simulink model "montagemrobo2"  (R2018a)
settings: Solver=VariableStepAuto  StartTime=0.0  StopTime=120  RelTol=1e-3
model workspace: external: MATLAB File C:\Users\Thiago\Documents\1- Faculdade\Robotica\2020.1\TRABALHO\simulink\montagemrobo_DataFile1.m (data not in the file)
values from neighbouring files (symbols this model uses):
  m = [207.61613 346.81729 366.65763 243.34094 10.76884 27.61521 3.40236]    [matlab.mat]
undefined symbols (not defined in the file or in its folder): smiData, X, Y, Z
libraries: sm_lib x61, nesl_utility x7
(part 2 of 2)

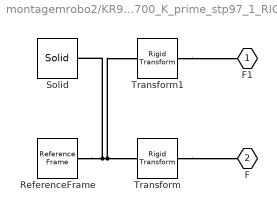
== system montagemrobo2/KR90_R3700_K_prime_stp97_1_RIGID ==
  ReferenceFrame : sm_lib/Frames and Transforms/Reference Frame
  Solid : sm_lib/Body Elements/Solid  InertiaType=Custom  Mass=smiData.Solid(6).mass  MassUnits=kg  CenterOfMass=smiData.Solid(6).CoM  CenterOfMassUnits=mm  MomentsOfInertia=smiData.Solid(6).MoI  MomentsOfInertiaUnits=kg*mm^2  ProductsOfInertia=smiData.Solid(6).PoI  ProductsOfInertiaUnits=kg*mm^2  DensityBased=on  Density=1000  DensityUnits=kg/m^3  DoExposeReferenceFrame=on  SerializedFrames=<Frames/>  GraphicType=FromGeometry  MarkerShape=Sphere  MarkerSize=10  GraphicVisPropType=SimpleVisualProperties  GraphicDiffuseColor=smiData.Solid(6).color  GraphicSpecularColor=[0.5 0.5 0.5 1.0]  GraphicAmbientColor=[0.15 0.15 0.15 1.0]  GraphicEmissiveColor=[0.0 0.0 0.0 1.0]  GraphicShininess=75  GraphicOpacity=smiData.Solid(6).opacity  GeometryShape=FromFile  RectangleSize=[1 1]  RectangleSizeUnits=m  BrickDimensions=[1 1 1]  BrickDimensionUnits=m  CylinderRadius=1  CylinderRadiusUnits=m  CylinderLength=1  CylinderLengthUnits=m  SphereRadius=1  SphereRadiusUnits=m  EllipsoidRadii=[1 1 1]  EllipsoidRadiiUnits=m  ExtrusionCrossSection=[1 1; -1 1; -1 -1; 1 -1]  ExtrusionCrossSectionUnits=m  ExtrusionLength=1  ExtrusionLengthUnits=m  PolygonNumSides=3  PolygonOuterRadius=1  PolygonOuterRadiusUnits=m  ExtGeomFileType=STEP  ExtGeomFileName=KR90_R3700_K_prime.stp[97]_Valor predeterminado_sldprt.STEP  ExtGeomFileUnits=m  RevolutionCrossSection=[1 1; 1 -1; 2 -1; 2 1]  RevolutionCrossSectionUnits=m  RevolutionExtent=Full  RevolutionAngle=180  RevolutionAngleUnits=deg
  Transform : sm_lib/Frames and Transforms/Rigid Transform  TranslationMethod=Cartesian  TranslationStandardOffset=0  TranslationLengthUnit=mm  TranslationStandardAxis=+Z  TranslationCartesianOffset=smiData.RigidTransform(4).translation  TranslationROffset=0  TranslationROffsetUnits=m  TranslationZOffset=0  TranslationZOffsetUnits=m  TranslationThetaOffset=0  TranslationThetaOffsetUnits=deg  RotationMethod=ArbitraryAxis  RotationAngleUnits=rad  RotationStandardAxis=+Z  RotationAngle=smiData.RigidTransform(4).angle  RotationArbitraryAxis=smiData.RigidTransform(4).axis  FollAlignAxisA=+X  BaseAlignAxisA=+Y  FollAlignAxisB=+Y  BaseAlignAxisB=+Z  RotationSequenceAxes=FollowerAxes  RotationSequence=XYX  RotationSequenceAngles=[0 0 0]  RotationSequenceAnglesUnits=deg  RotationMatrix=[1 0 0; 0 1 0; 0 0 1]
  Transform1 : sm_lib/Frames and Transforms/Rigid Transform  TranslationMethod=Cartesian  TranslationStandardOffset=0  TranslationLengthUnit=mm  TranslationStandardAxis=+Z  TranslationCartesianOffset=smiData.RigidTransform(12).translation  TranslationROffset=0  TranslationROffsetUnits=m  TranslationZOffset=0  TranslationZOffsetUnits=m  TranslationThetaOffset=0  TranslationThetaOffsetUnits=deg  RotationMethod=ArbitraryAxis  RotationAngleUnits=rad  RotationStandardAxis=+Z  RotationAngle=smiData.RigidTransform(12).angle  RotationArbitraryAxis=smiData.RigidTransform(12).axis  FollAlignAxisA=+X  BaseAlignAxisA=+Y  FollAlignAxisB=+Y  BaseAlignAxisB=+Z  RotationSequenceAxes=FollowerAxes  RotationSequence=XYX  RotationSequenceAngles=[0 0 0]  RotationSequenceAnglesUnits=deg  RotationMatrix=[1 0 0; 0 1 0; 0 0 1]
  F1 : PMIOPort  Side=Right
  F : PMIOPort  Port=2  Side=Left
  connections:
  Solid/RConn1 -- ReferenceFrame/RConn1 -- Transform/LConn1 -- Transform1/LConn1
  Transform/RConn1 -- F/RConn1
  Transform1/RConn1 -- F1/RConn1

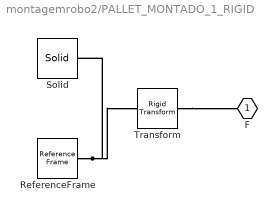
== system montagemrobo2/PALLET_MONTADO_1_RIGID ==
  ReferenceFrame : sm_lib/Frames and Transforms/Reference Frame
  Solid : sm_lib/Body Elements/Solid  InertiaType=Custom  Mass=smiData.Solid(2).mass  MassUnits=kg  CenterOfMass=smiData.Solid(2).CoM  CenterOfMassUnits=mm  MomentsOfInertia=smiData.Solid(2).MoI  MomentsOfInertiaUnits=kg*mm^2  ProductsOfInertia=smiData.Solid(2).PoI  ProductsOfInertiaUnits=kg*mm^2  DensityBased=on  Density=1000  DensityUnits=kg/m^3  DoExposeReferenceFrame=on  SerializedFrames=<Frames/>  GraphicType=FromGeometry  MarkerShape=Sphere  MarkerSize=10  GraphicVisPropType=SimpleVisualProperties  GraphicDiffuseColor=smiData.Solid(2).color  GraphicSpecularColor=[0.5 0.5 0.5 1.0]  GraphicAmbientColor=[0.15 0.15 0.15 1.0]  GraphicEmissiveColor=[0.0 0.0 0.0 1.0]  GraphicShininess=75  GraphicOpacity=smiData.Solid(2).opacity  GeometryShape=FromFile  RectangleSize=[1 1]  RectangleSizeUnits=m  BrickDimensions=[1 1 1]  BrickDimensionUnits=m  CylinderRadius=1  CylinderRadiusUnits=m  CylinderLength=1  CylinderLengthUnits=m  SphereRadius=1  SphereRadiusUnits=m  EllipsoidRadii=[1 1 1]  EllipsoidRadiiUnits=m  ExtrusionCrossSection=[1 1; -1 1; -1 -1; 1 -1]  ExtrusionCrossSectionUnits=m  ExtrusionLength=1  ExtrusionLengthUnits=m  PolygonNumSides=3  PolygonOuterRadius=1  PolygonOuterRadiusUnits=m  ExtGeomFileType=STEP  ExtGeomFileName=PALLET.MONTADO_Valor predeterminado_sldprt.STEP  ExtGeomFileUnits=m  RevolutionCrossSection=[1 1; 1 -1; 2 -1; 2 1]  RevolutionCrossSectionUnits=m  RevolutionExtent=Full  RevolutionAngle=180  RevolutionAngleUnits=deg
  Transform : sm_lib/Frames and Transforms/Rigid Transform  TranslationMethod=Cartesian  TranslationStandardOffset=0  TranslationLengthUnit=mm  TranslationStandardAxis=+Z  TranslationCartesianOffset=smiData.RigidTransform(15).translation  TranslationROffset=0  TranslationROffsetUnits=m  TranslationZOffset=0  TranslationZOffsetUnits=m  TranslationThetaOffset=0  TranslationThetaOffsetUnits=deg  RotationMethod=ArbitraryAxis  RotationAngleUnits=rad  RotationStandardAxis=+Z  RotationAngle=smiData.RigidTransform(15).angle  RotationArbitraryAxis=smiData.RigidTransform(15).axis  FollAlignAxisA=+X  BaseAlignAxisA=+Y  FollAlignAxisB=+Y  BaseAlignAxisB=+Z  RotationSequenceAxes=FollowerAxes  RotationSequence=XYX  RotationSequenceAngles=[0 0 0]  RotationSequenceAnglesUnits=deg  RotationMatrix=[1 0 0; 0 1 0; 0 0 1]
  F : PMIOPort  Side=Left
  connections:
  Solid/RConn1 -- ReferenceFrame/RConn1 -- Transform/LConn1
  Transform/RConn1 -- F/RConn1

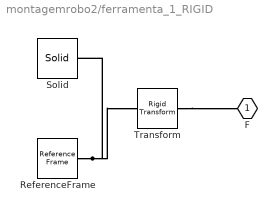
== system montagemrobo2/ferramenta_1_RIGID ==
  ReferenceFrame : sm_lib/Frames and Transforms/Reference Frame
  Solid : sm_lib/Body Elements/Solid  InertiaType=Custom  Mass=smiData.Solid(10).mass  MassUnits=kg  CenterOfMass=smiData.Solid(10).CoM  CenterOfMassUnits=mm  MomentsOfInertia=smiData.Solid(10).MoI  MomentsOfInertiaUnits=kg*mm^2  ProductsOfInertia=smiData.Solid(10).PoI  ProductsOfInertiaUnits=kg*mm^2  DensityBased=on  Density=1000  DensityUnits=kg/m^3  DoExposeReferenceFrame=on  SerializedFrames=<Frames/>  GraphicType=FromGeometry  MarkerShape=Sphere  MarkerSize=10  GraphicVisPropType=SimpleVisualProperties  GraphicDiffuseColor=smiData.Solid(10).color  GraphicSpecularColor=[0.5 0.5 0.5 1.0]  GraphicAmbientColor=[0.15 0.15 0.15 1.0]  GraphicEmissiveColor=[0.0 0.0 0.0 1.0]  GraphicShininess=75  GraphicOpacity=smiData.Solid(10).opacity  GeometryShape=FromFile  RectangleSize=[1 1]  RectangleSizeUnits=m  BrickDimensions=[1 1 1]  BrickDimensionUnits=m  CylinderRadius=1  CylinderRadiusUnits=m  CylinderLength=1  CylinderLengthUnits=m  SphereRadius=1  SphereRadiusUnits=m  EllipsoidRadii=[1 1 1]  EllipsoidRadiiUnits=m  ExtrusionCrossSection=[1 1; -1 1; -1 -1; 1 -1]  ExtrusionCrossSectionUnits=m  ExtrusionLength=1  ExtrusionLengthUnits=m  PolygonNumSides=3  PolygonOuterRadius=1  PolygonOuterRadiusUnits=m  ExtGeomFileType=STEP  ExtGeomFileName=ferramenta_Valor predeterminado_sldprt.STEP  ExtGeomFileUnits=m  RevolutionCrossSection=[1 1; 1 -1; 2 -1; 2 1]  RevolutionCrossSectionUnits=m  RevolutionExtent=Full  RevolutionAngle=180  RevolutionAngleUnits=deg
  Transform : sm_lib/Frames and Transforms/Rigid Transform  TranslationMethod=Cartesian  TranslationStandardOffset=0  TranslationLengthUnit=mm  TranslationStandardAxis=+Z  TranslationCartesianOffset=smiData.RigidTransform(18).translation  TranslationROffset=0  TranslationROffsetUnits=m  TranslationZOffset=0  TranslationZOffsetUnits=m  TranslationThetaOffset=0  TranslationThetaOffsetUnits=deg  RotationMethod=ArbitraryAxis  RotationAngleUnits=rad  RotationStandardAxis=+Z  RotationAngle=smiData.RigidTransform(18).angle  RotationArbitraryAxis=smiData.RigidTransform(18).axis  FollAlignAxisA=+X  BaseAlignAxisA=+Y  FollAlignAxisB=+Y  BaseAlignAxisB=+Z  RotationSequenceAxes=FollowerAxes  RotationSequence=XYX  RotationSequenceAngles=[0 0 0]  RotationSequenceAnglesUnits=deg  RotationMatrix=[1 0 0; 0 1 0; 0 0 1]
  F : PMIOPort  Side=Left
  connections:
  Solid/RConn1 -- ReferenceFrame/RConn1 -- Transform/LConn1
  Transform/RConn1 -- F/RConn1

== matlab function montagemrobo2/MATLAB Function1 ==
  data: tarefa input; valor_q_inv output; t input
function valor_q_inv  = cinematica(tarefa,t)

%clear all, clc, close all
%% 
%   Rotina para cálculo da cinemática direta e inversa de um manipulador
%   antropomórfico alterada para robô da tarefa do estoque
%
%   Autor:  Luciano
%   Data:   09-11-2020
%
%   Revisão: Grupo
%   Data:    06-01-2021

% %% Definição de variáveis
% 
% syms q1 q2 q3 q4 q5 q6
% 
% q = [q1; q2; q3; q4; q5; q6];
% 
% syms dq1 dq2 dq3 dq4 dq5 dq6
% 
% dq = [dq1; dq2; dq3; dq4; dq5; dq6];
% 
% syms d2q1 d2q2 d2q3 d2q4 d2q5 d2q6
% 
% d2q = [d2q1; d2q2; d2q3; d2q4; d2q5; d2q6];
% 
% syms L1 L2 L3 L4 
% 
% syms E1 E2                          %excentricidades e1=750; e2=-41
% 
% syms xf yf zf
% 
% syms xG1 yG1 zG1 xG2 yG2 zG2 xG3 yG3 zG3 xG4 yG4 zG4 xG5 yG5 zG5 xG6 yG6 zG6 xGf yGf zGf
% 
% syms xC yC zC qxC qyC qzC
% 
% syms x7_C y7_C z7_C alfa beta phi

xC = 0; yC = 0; zC = 0; qxC = 0; qyC = 0; qzC = 0; 
%alfa = 0; beta = 0; phi = 0;
L1=0.590; L2=1.350;L3=1.600;L4=0.215;
xf=0.22485;yf=0;zf=0;
E1=0.750; E2=-0.041;
q_possiveis=zeros(20,6);
x7_C=tarefa(1);
y7_C=tarefa(2);
z7_C=tarefa(3);
phi=tarefa(4);
beta=tarefa(5);
alfa=tarefa(6);





% %% Análise do Elo 1
% R1_0 = [cos(q1) -sin(q1) 0 0; sin(q1) cos(q1) 0 0; 0 0 1 0; 0 0 0 1];
% D1_0 = [1 0 0 E1; 0 1 0 0; 0 0 1 L1; 0 0 0 1];
% T1_0 = R1_0*D1_0;
% p1_0 = T1_0(1:3,4);
% JL1_0 = jacobian(p1_0,q);
% v1_0 = JL1_0*dq;
% dJL1_0 = [jacobian(JL1_0(:,1),q)*dq jacobian(JL1_0(:,2),q)*dq jacobian(JL1_0(:,3),q)*dq jacobian(JL1_0(:,4),q)*dq jacobian(JL1_0(:,5),q)*dq jacobian(JL1_0(:,6),q)*dq];
% a1_0 = JL1_0*d2q + dJL1_0*dq;
% 
% JA1_0 = [T1_0(1:3,3) zeros(3,5)];
% w1_0 = JA1_0*dq;
% dJA1_0 = [jacobian(JA1_0(:,1),q)*dq jacobian(JA1_0(:,2),q)*dq jacobian(JA1_0(:,3),q)*dq jacobian(JA1_0(:,4),q)*dq jacobian(JA1_0(:,5),q)*dq jacobian(JA1_0(:,6),q)*dq];
% dw1_0 = JA1_0*d2q + dJA1_0*dq;
% 
% pG1_1 = [xG1; yG1; zG1; 1];
% aux = T1_0*pG1_1;
% pG1_0 = aux(1:3,1);
% JLG1_0 = jacobian(pG1_0,q);
% vG1_0 = JLG1_0*dq;
% dJLG1_0 = [jacobian(JLG1_0(:,1),q)*dq jacobian(JLG1_0(:,2),q)*dq jacobian(JLG1_0(:,3),q)*dq jacobian(JLG1_0(:,4),q)*dq jacobian(JLG1_0(:,5),q)*dq jacobian(JLG1_0(:,6),q)*dq];
% aG1_0 = JLG1_0*d2q + dJLG1_0*dq;
% 
% %% Análise do Elo 2
% R2_1 = [cos(q2) 0 sin(q2) 0; 0 1 0 0; -sin(q2) 0 cos(q2) 0; 0 0 0 1];
% D2_1 = [1 0 0 L2; 0 1 0 0; 0 0 1 E2; 0 0 0 1];
% T2_1 = R2_1*D2_1;
% T2_0 = T1_0*T2_1;
% p2_0 = T2_0(1:3,4);
% JL2_0 = jacobian(p2_0,q);
% v2_0 = JL2_0*dq;
% dJL2_0 = [jacobian(JL2_0(:,1),q)*dq jacobian(JL2_0(:,2),q)*dq jacobian(JL2_0(:,3),q)*dq jacobian(JL2_0(:,4),q)*dq jacobian(JL2_0(:,5),q)*dq jacobian(JL2_0(:,6),q)*dq];
% a2_0 = simplify(JL2_0*d2q + dJL2_0*dq);
% 
% JA2_0 = [T1_0(1:3,3) T2_0(1:3,2) zeros(3,4)];
% w2_0 = JA2_0*dq;
% dJA2_0 = [jacobian(JA2_0(:,1),q)*dq jacobian(JA2_0(:,2),q)*dq jacobian(JA2_0(:,3),q)*dq jacobian(JA2_0(:,4),q)*dq jacobian(JA2_0(:,5),q)*dq jacobian(JA2_0(:,6),q)*dq];
% dw2_0 = JA2_0*d2q + dJA2_0*dq;
% 
% pG2_2 = [xG2; yG2; zG2; 1];
% aux = T2_0*pG2_2;
% pG2_0 = aux(1:3,1);
% JLG2_0 = jacobian(pG2_0,q);
% vG2_0 = JLG2_0*dq;
% dJLG2_0 = [jacobian(JLG2_0(:,1),q)*dq jacobian(JLG2_0(:,2),q)*dq jacobian(JLG2_0(:,3),q)*dq jacobian(JLG2_0(:,4),q)*dq jacobian(JLG2_0(:,5),q)*dq jacobian(JLG2_0(:,6),q)*dq];
% aG2_0 = JLG2_0*d2q + dJLG2_0*dq;
% 
% %% Análise do Elo 3
% R3_2 = [cos(q3) 0 sin(q3) 0; 0 1 0 0; -sin(q3) 0 cos(q3) 0; 0 0 0 1];
% D3_2 = [1 0 0 L3; 0 1 0 0; 0 0 1 0; 0 0 0 1];
% T3_2 = R3_2*D3_2;
% T3_0 = simplify(T2_0*T3_2);
% p3_0 = T3_0(1:3,4);
% JL3_0 = jacobian(p3_0,q);
% v3_0 = JL3_0*dq;
% dJL3_0 = [jacobian(JL3_0(:,1),q)*dq jacobian(JL3_0(:,2),q)*dq jacobian(JL3_0(:,3),q)*dq jacobian(JL3_0(:,4),q)*dq jacobian(JL3_0(:,5),q)*dq jacobian(JL3_0(:,6),q)*dq];
% a3_0 = simplify(JL3_0*d2q + dJL3_0*dq);
% 
% JA3_0 = [T1_0(1:3,3) T2_0(1:3,2) T3_0(1:3,2) zeros(3,3)];
% w3_0 = JA3_0*dq;
% dJA3_0 = [jacobian(JA3_0(:,1),q)*dq jacobian(JA3_0(:,2),q)*dq jacobian(JA3_0(:,3),q)*dq jacobian(JA3_0(:,4),q)*dq jacobian(JA3_0(:,5),q)*dq jacobian(JA3_0(:,6),q)*dq];
% dw3_0 = JA3_0*d2q + dJA3_0*dq;
% 
% pG3_3 = [xG3; yG3; zG3; 1];
% aux = T3_0*pG3_3;
% pG3_0 = aux(1:3,1);
% JLG3_0 = jacobian(pG3_0,q);
% vG3_0 = JLG3_0*dq;
% dJLG3_0 = [jacobian(JLG3_0(:,1),q)*dq jacobian(JLG3_0(:,2),q)*dq jacobian(JLG3_0(:,3),q)*dq jacobian(JLG3_0(:,4),q)*dq jacobian(JLG3_0(:,5),q)*dq jacobian(JLG3_0(:,6),q)*dq];
% aG3_0 = JLG3_0*d2q + dJLG3_0*dq;
% 
% %% Análiose do Elo 4
% R4_3 = [1 0 0 0; 0 cos(q4) -sin(q4) 0; 0 sin(q4) cos(q4) 0; 0 0 0 1];
% T4_3 = R4_3;
% T4_0 = simplify(T3_0*T4_3);
% p4_0 = p3_0;
% JL4_0 = JL3_0;
% v4_0 = v3_0;
% dJL4_0 = dJL3_0;
% a4_0 = a3_0;
% 
% JA4_0 = [T1_0(1:3,3) T2_0(1:3,2) T3_0(1:3,2) T4_0(1:3,1) zeros(3,2)];
% w4_0 = JA4_0*dq;
% dJA4_0 = [jacobian(JA4_0(:,1),q)*dq jacobian(JA4_0(:,2),q)*dq jacobian(JA4_0(:,3),q)*dq jacobian(JA4_0(:,4),q)*dq jacobian(JA4_0(:,5),q)*dq jacobian(JA4_0(:,6),q)*dq];
% dw4_0 = JA4_0*d2q + dJA4_0*dq;
% 
% pG4_4 = [xG4; yG4; zG4; 1];
% aux = T4_0*pG4_4;
% pG4_0 = aux(1:3,1);
% JLG4_0 = jacobian(pG4_0,q);
% vG4_0 = JLG4_0*dq;
% dJLG4_0 = [jacobian(JLG4_0(:,1),q)*dq jacobian(JLG4_0(:,2),q)*dq jacobian(JLG4_0(:,3),q)*dq jacobian(JLG4_0(:,4),q)*dq jacobian(JLG4_0(:,5),q)*dq jacobian(JLG4_0(:,6),q)*dq];
% aG4_0 = JLG4_0*d2q + dJLG4_0*dq;
% 
% %% Análise do Elo 5
% R5_4 = [cos(q5) 0 sin(q5) 0; 0 1 0 0; -sin(q5) 0 cos(q5) 0; 0 0 0 1];
% T5_4 = R5_4;
% T5_0 = simplify(T4_0*T5_4);
% p5_0 = p4_0;
% JL5_0 = JL4_0;
% v5_0 = v4_0;
% dJL5_0 = dJL4_0;
% a5_0 = a4_0;
% 
% JA5_0 = [T1_0(1:3,3) T2_0(1:3,2) T3_0(1:3,2) T4_0(1:3,1) T5_0(1:3,2) zeros(3,1)];
% w5_0 = JA5_0*dq;
% dJA5_0 = [jacobian(JA5_0(:,1),q)*dq jacobian(JA5_0(:,2),q)*dq jacobian(JA5_0(:,3),q)*dq jacobian(JA5_0(:,4),q)*dq jacobian(JA5_0(:,5),q)*dq jacobian(JA5_0(:,6),q)*dq];
% dw5_0 = JA5_0*d2q + dJA5_0*dq;
% 
% pG5_5 = [xG5; yG5; zG5; 1];
% aux = T5_0*pG5_5;
% pG5_0 = aux(1:3,1);
% JLG5_0 = jacobian(pG5_0,q);
% vG5_0 = JLG5_0*dq;
% dJLG5_0 = [jacobian(JLG5_0(:,1),q)*dq jacobian(JLG5_0(:,2),q)*dq jacobian(JLG5_0(:,3),q)*dq jacobian(JLG5_0(:,4),q)*dq jacobian(JLG5_0(:,5),q)*dq jacobian(JLG5_0(:,6),q)*dq];
% aG5_0 = JLG5_0*d2q + dJLG5_0*dq;
% 
% %% Análise do Elo 6
% R6_5 = [1 0 0 0; 0 cos(q6) -sin(q6) 0; 0 sin(q6) cos(q6) 0; 0 0 0 1];
% T6_5 = R6_5;
% T6_0 = simplify(T5_0*T6_5);
% T6_3 = simplify(T4_3*T5_4*T6_5);
% p6_0 = p5_0;
% JL6_0 = JL5_0;
% v6_0 = v5_0;
% dJL6_0 = dJL5_0;
% a6_0 = a5_0;
% 
% JA6_0 = [T1_0(1:3,3) T2_0(1:3,2) T3_0(1:3,2) T4_0(1:3,1) T5_0(1:3,2) T6_0(1:3,1)];
% w6_0 = JA6_0*dq;
% dJA6_0 = [jacobian(JA6_0(:,1),q)*dq jacobian(JA6_0(:,2),q)*dq jacobian(JA6_0(:,3),q)*dq jacobian(JA6_0(:,4),q)*dq jacobian(JA6_0(:,5),q)*dq jacobian(JA6_0(:,6),q)*dq];
% dw6_0 = JA6_0*d2q + dJA6_0*dq;
% 
% pG6_6 = [xG6; yG6; zG6; 1];
% aux = T6_0*pG6_6;
% pG6_0 = aux(1:3,1);
% JLG6_0 = jacobian(pG6_0,q);
% vG6_0 = JLG6_0*dq;
% dJLG6_0 = [jacobian(JLG6_0(:,1),q)*dq jacobian(JLG6_0(:,2),q)*dq jacobian(JLG6_0(:,3),q)*dq jacobian(JLG6_0(:,4),q)*dq jacobian(JLG6_0(:,5),q)*dq jacobian(JLG6_0(:,6),q)*dq];
% aG6_0 = JLG6_0*d2q + dJLG6_0*dq;
% 
% %% Análise do Ferramenta
 D7_6 = [1 0 0 L4+xf; 0 1 0 yf; 0 0 1 zf; 0 0 0 1];
 T7_6 = D7_6;
%T7_0 = simplify(T6_0*T7_6);
% p7_0 = T7_0(1:3,4);
% JL7_0 = jacobian(p7_0,q);
% v7_0 = simplify(JL7_0*dq);
% dJL7_0 = [jacobian(JL7_0(:,1),q)*dq jacobian(JL7_0(:,2),q)*dq jacobian(JL7_0(:,3),q)*dq jacobian(JL7_0(:,4),q)*dq jacobian(JL7_0(:,5),q)*dq jacobian(JL7_0(:,6),q)*dq];
% a7_0 = simplify(JL7_0*d2q + dJL7_0*dq);
% 
% w7_0 = w6_0;
% dw7_0 = dw6_0;
% 
% pG7_7 = [xGf; yGf; zGf; 1];
% aux = T7_0*pG7_7;
% pG7_0 = aux(1:3,1);
% JLG7_0 = jacobian(pG7_0,q);
% vG7_0 = JLG7_0*dq;
% dJLG7_0 = [jacobian(JLG7_0(:,1),q)*dq jacobian(JLG7_0(:,2),q)*dq jacobian(JLG7_0(:,3),q)*dq jacobian(JLG7_0(:,4),q)*dq jacobian(JLG7_0(:,5),q)*dq jacobian(JLG7_0(:,6),q)*dq];
% aG7_0 = JLG7_0*d2q + dJLG7_0*dq;

%% Parametrização da tarefa x ferramenta

% Definição do ambiente de trabalho
DC_0 = [1 0 0 xC; 0 1 0 yC; 0 0 1 zC; 0 0 0 1];
Rz_qzC = [cos(qzC) -sin(qzC) 0 0; sin(qzC) cos(qzC) 0 0; 0 0 1 0; 0 0 0 1];
Ry_qyC = [cos(qyC) 0 sin(qyC) 0; 0 1 0 0; -sin(qyC) 0 cos(qyC) 0; 0 0 0 1];
Rx_qxC = [1 0 0 0; 0 cos(qxC) -sin(qxC) 0; 0 sin(qxC) cos(qxC) 0; 0 0 0 1];
RC_0 = Rz_qzC*Ry_qyC*Rx_qxC;
TC_0 = DC_0*RC_0;
% 
% Tarefa
D7_C = [1 0 0 x7_C; 0 1 0 y7_C; 0 0 1 z7_C; 0 0 0 1];
Rz_alfa = [cos(alfa) -sin(alfa) 0 0; sin(alfa) cos(alfa) 0 0; 0 0 1 0; 0 0 0 1];
Ry_beta = [cos(beta) 0 sin(beta) 0; 0 1 0 0; -sin(beta) 0 cos(beta) 0; 0 0 0 1];
Rx_phi = [1 0 0 0; 0 cos(phi) -sin(phi) 0; 0 sin(phi) cos(phi) 0; 0 0 0 1];
R7_C = Rz_alfa*Ry_beta*Rx_phi;
T7_C = D7_C*R7_C;

% Juntar tarefa e ambiente
T7_0f = TC_0*T7_C;
R7_0f = RC_0*R7_C;

% % xC = 1; yC = 1; zC = 0.7; qxC = 0; qyC = 0; qzC = 0; 
% % x7_C = 0; y7_C = 0; z7_C = 0; alfa = 0; beta = pi/2; phi = 0;
% % aux = eval(T7_0f)
% 
%% Definição da posição do pulso no referencial da base do robô - {0}
p7_0f = T7_0f(1:3,4);
p3_7_7f = [-L4-xf; -yf; -zf; 1];
aux = R7_0f*p3_7_7f;
p3_0f = p7_0f + aux(1:3,1);
% 
% return
% %% Simulações


%% INVERSA || PARTE 1 q possiveis

%%%% Variaveis a receber %%%%%%%%%
%P3_0f <- numerico
%T3_0 <- ou criar dentro 
%T6_3 <- ou criar dentro
%T7_0f <- ou criar dentro ||  Problema se manter L4+E2 no T7_6  
%
%%%%%%%%%%%%%%%%%%
%%%%%%%%%q_possiveis=zeros(10,6); Testar se necessita ou pode apagar
X=p3_0f(1);
Y=p3_0f(2);
Z=p3_0f(3);
ind_k=0;
q1=atan2(Y,X);
if isreal(q1)==0
    error("Região fora da area de trabalho");
end
%if q1>deg2rad(185) || q1<deg2rad(-185)
%    error("Região fora da area de trabalho");
%end

if sin(q1)<0.1 && sin(q1)>-0.1
    aux=X/cos(q1);
    
else
    aux=Y/sin(q1);
    
end


%- 2*L1*zC  + E2^2+ L2^2 + aux^2 + E1^2 + L1^2 + zC^2 + 2*L2*zC*sin(q2) - (2*E1)*aux + 2*E1*L2*cos(q2) + 2*E2*L1*cos(q2) + 2*E1*E2*sin(q2) - 2*L1*L2*sin(q2) - 2*E2*zC*cos(q2) - (2*L2*cos(q2)*aux) - (2*E2*sin(q2))*aux-L3^2

           



A_q2=2*E1*L2-2*aux*L2;
B_q2=2*Z*L2-2*L1*L2;
C_q2=L2^2+E1^2-2*E1*aux-2*Z*L1+Z^2-E2^2-L3^2+aux^2+L1^2;

delta_q2= 4*A_q2^2*C_q2^2-4*(A_q2^2+B_q2^2)*(C_q2^2-B_q2^2);
if delta_q2<0
    error("Fora da região de trabalho");
end

 
 q2a=zeros(1,4);
 argumanq2a1=((-2*A_q2*C_q2+sqrt(delta_q2))/(2*(A_q2^2+B_q2^2)));
 argumanq2a1 = max(min(argumanq2a1,1),-1);
 
 argumanq2a2=((-2*A_q2*C_q2-sqrt(delta_q2))/(2*(A_q2^2+B_q2^2)));
 argumanq2a2 = max(min(argumanq2a2,1),-1);
 
 q2a(1)=acos(argumanq2a1);
 q2a(2)=acos(argumanq2a2);
 q2a(3)=-q2a(1);
 q2a(4)=-q2a(2);

%%%%%% PARTE NOVA %%%%%%%%%%%%%%%%%%%%
q3a=zeros(1,4);
for i=1:1:4 %valores q2
    q2=q2a(i);
    if q2>deg2rad(-120) && q2<deg2rad(70) && isreal(q2)==1
        %colocar bloco de restrição de altura se a tarefa requirir | if altura > blablabla continue%
     A_q3=E2*cos(q2)-L3*sin(q2);
     B_q3=-L3*cos(q2)-E2*sin(q2);
     C_q3=L1-L2*sin(q2)-Z;
     delta_q3= 4*A_q3^2*C_q3^2-4*(A_q3^2+B_q3^2)*(C_q3^2-B_q3^2);
     if delta_q3 < 0
         continue
     end
     
      argumanq3a1=((-2*A_q3*C_q3+sqrt(delta_q3))/(2*(A_q3^2+B_q3^2)));
      argumanq3a1 = max(min(argumanq3a1,1),-1);
 
      argumanq3a2=((-2*A_q3*C_q3-sqrt(delta_q3))/(2*(A_q3^2+B_q3^2)));
      argumanq3a2 = max(min(argumanq3a2,1),-1);
     

     q3a(1)=acos(argumanq3a1);
     q3a(2)=acos(argumanq3a2);
     q3a(3)=-q3a(1);
     q3a(4)=-q3a(2);
        for i2=1:1:4 %valores q3
            q3=q3a(i2);
            if q3>deg2rad(-120) && q3<deg2rad(155) && isreal(q3)==1
                R1_0 = [cos(q1) -sin(q1) 0 0; sin(q1) cos(q1) 0 0; 0 0 1 0; 0 0 0 1];
                D1_0 = [1 0 0 E1; 0 1 0 0; 0 0 1 L1; 0 0 0 1];
                T1_0 = R1_0*D1_0;
                R2_1 = [cos(q2) 0 sin(q2) 0; 0 1 0 0; -sin(q2) 0 cos(q2) 0; 0 0 0 1];
                D2_1 = [1 0 0 L2; 0 1 0 0; 0 0 1 0; 0 0 0 1];
                T2_1 = R2_1*D2_1;
                T2_0 = T1_0*T2_1;
                R3_2 = [cos(q3) 0 sin(q3) 0; 0 1 0 0; -sin(q3) 0 cos(q3) 0; 0 0 0 1];
                D3_2 = [1 0 0 L3; 0 1 0 0; 0 0 1 E2; 0 0 0 1];
                T3_2 = R3_2*D3_2;
                T3_0 = T2_0*T3_2;
                T3_0num=T3_0;
                if norm(T3_0num(1,4)-X)<0.0001 && norm(T3_0num(2,4)-Y)<0.0001 && norm(T3_0num(3,4)-Z) <0.0001 %opcional
                    T6_0fnum=T7_0f*inv(T7_6); %%%% SE VIER DE OUTRO BLOCO VIRA NUMERICA
                    T6_3num=inv(T3_0num)*T6_0fnum; %%% COMPARAR COM T6_3
                    q4=atan2(T6_3num(2,1),-T6_3num(3,1)); %% q4 estara sempre no intervalo [-350;350] graus devido a funcao atan2
                    q6=atan2(T6_3num(1,2),T6_3num(1,3)); %% iden a q4 sobre o intervalo
                    q5a=zeros(1,2);
                    q5a(1)=acos(T6_3num(1,1));
                    q5a(2)=-q5a(1);
                    if isreal(q4) == 1 && isreal(q6) == 1 %q4 e q6 reais
                        for i3=1:1:2 %valores q5
                            if q5a(i3)>deg2rad(-125) && q5a(i3)<deg2rad(125) && isreal(q5a) ==1 %q5 valido
                                q5=q5a(i3);
                                 R4_3 = [1 0 0 0; 0 cos(q4) -sin(q4) 0; 0 sin(q4) cos(q4) 0; 0 0 0 1];
                                 T4_3 = R4_3;
                                 T4_0 =T3_0*T4_3;
                                 R5_4 = [cos(q5) 0 sin(q5) 0; 0 1 0 0; -sin(q5) 0 cos(q5) 0; 0 0 0 1];
                                 T5_4 = R5_4;
                                 T5_0 = T4_0*T5_4;                               
                                 R6_5 = [1 0 0 0; 0 cos(q6) -sin(q6) 0; 0 sin(q6) cos(q6) 0; 0 0 0 1];
                                 T6_5 = R6_5;
                                 T6_0 = T5_0*T6_5;                               
                                T7_0num=T6_0*T7_6;
                                if norm(T7_0num(1,4)-p7_0f(1))<0.0001 && norm(T7_0num(2,4)-p7_0f(2))<0.0001 && norm(T7_0num(3,4)-p7_0f(3))<0.0001
                                    ind_k=ind_k+1;
                                    q_possiveis(ind_k,1)=q1;
                                    q_possiveis(ind_k,2)=q2;
                                    q_possiveis(ind_k,3)=q3;
                                    q_possiveis(ind_k,4)=q4;
                                    q_possiveis(ind_k,5)=q5;
                                    q_possiveis(ind_k,6)=q6;
                                end %pos braço valida
                            end %if q5 valido
                        end %valores q5                
                    end %q4 e q6 validos
                end %checar posicao braco
            end %q3 validos
        end %valores q3
    end % q2 validos
end %valores q2

% PARTE 2 , pegar combinacao de q mais proxima da anterior
coder.extrinsic('evalin')
coder.extrinsic('assignin')
menor_desloc=0;
if t==0
    Qs=[0 0 0 0 0 0]; %%%POSIÇÃO INICIAL ESTÁ CERTA ?
else
    Qs=evalin('caller','Qs');
end
valor_q_inv=zeros(1,6);
%fprintf("Realizando inversa do ponto %d\n",ind_ponto)
%[q_possiveis,ind_k]=inversa_q_possiveis(mat71);
if ind_k<1
   error("ERRO: Naoo foi possivel realizar uma movimentacao para o ponto")
end
for z=1:ind_k
    vetor_deslocamento_ang=q_possiveis(z,:)-Qs;
    if z==1
        menor_desloc=norm(vetor_deslocamento_ang);
        valor_q_inv=q_possiveis(z,:);
    else
        if norm(vetor_deslocamento_ang) < menor_desloc
            valor_q_inv=q_possiveis(z,:);
            menor_desloc=norm(vetor_deslocamento_ang);
        end
    end
end
assignin('base','Qs',valor_q_inv);

== matlab function montagemrobo2/MATLAB Function ==
  data: t input; tarefa output

function tarefa = trajetoria(t)
X=0;
Y=2500;
Z=950;
alfa=0;
beta=0;
gama=0;

if t>=0 && t<3 % Inicial -> Ponto de espera
%     X=coordenadas_pol( 0,0,t-3,3);
%     Y=coordenadas_pol(2050.15,2500,t-3,3);
%     Z=907.64;
%     alfa=0;
%     beta=0;
X=0;
Y=2500;
Z=950;
    gama=coordenadas_pol(0, deg2rad(90),t,3);
end

if t>=3 && t<6 %Ponto de espera -> caixa
    X=coordenadas_pol( 0,0,t-3,3);
    Y=coordenadas_pol(2050.15,2500,t-3,3);
    Z=907.64;
    alfa=0;
    beta=0;
    gama=deg2rad(90);
end

 if t>=6 && t<9 %Caixa -> ponto de espera
    X=0;
    Y=coordenadas_pol(2500,2050.15,t-6,3);
    Z=907.64;
    alfa=0;
    beta=0;
    gama=deg2rad(90);
 end
    
if t>=9 && t<15 %Ponto de espera -> Pos circuferencia
    raio=2050.15; 
    %pos_final_traj=-2040.39;
    %ang_final_traj=abs(acos(pos_final_traj/raio_traj));
    ang_final_traj=3.044;
    ang_inicial_traj=0;
    angulo=coordenadas_pol(ang_inicial_traj,ang_final_traj,t-9,6);
    Y=cos(angulo)*raio;
    X=sin(angulo)*raio;
    Z=907.64;
    alfa=0;
    beta=0;
    gama=coordenadas_pol(deg2rad(90),deg2rad(-90),t-9,6);
end

if t>=15 && t <18 % Pos circuferencia -> 10mm pallete
    X=coordenadas_pol(199.7621,199.85,t-15,3);
    Y=coordenadas_pol(-2040.39,-2049.85,t-15,3);
    Z=coordenadas_pol(907.64,255.64,t-15,3);
    alfa=0;
    beta=0;
    gama=deg2rad(-90);
end
    
if t>=18 && t<20 %10mm do pallete -> encaixe pallete
    X=199.85;
    Y=-2049.85;
    Z=coordenadas_pol(255.64,245.64,t-18,2);
    alfa=0;
    beta=0;
    gama=deg2rad(-90);
end
    
    
if t>=20 && t<22 % Encaixe pallete -> retraido Y caixa
    X=199.85;
    Y=coordenadas_pol(-2049.85,-1899.85,t-20,2);
    Z=245.64;
    alfa=0;
    beta=0;
    gama=deg2rad(-90);
end
    
if t>=22 && t<25 %Retraido caixa -> pos circuferencia
    X=coordenadas_pol(199.85,199.7621,t-22,3);
    Y=coordenadas_pol(-1899.85,-2040.39,t-22,3);
    Z=coordenadas_pol(245.64,907.64,t-22,3);
    alfa=0;
    beta=0;
    gama=deg2rad(-90);
end 
    
if t>=25 && t<31 %Pos circuferencia -> ponto de espera
    raio=2050.15; 
    ang_inicial_traj=3.044;
    ang_final_traj=0;
    angulo=coordenadas_pol(ang_inicial_traj,ang_final_traj,t-25,6);
    Y=cos(angulo)*raio;
    X=sin(angulo)*raio;
    Z=907.64;
    alfa=0;
    beta=0;
    gama=coordenadas_pol(deg2rad(-90),deg2rad(90),t-25,6);
end 
    
if t>=31 && t<34 %Ponto de espera -> Pegar caixa
    X=coordenadas_pol( 0,0,t-31,3);
    Y=coordenadas_pol(2050.15,2500,t-31,3);
    Z=907.64;
    alfa=0;
    beta=0;
    gama=deg2rad(90);
end 
    
if t>=34 && t<37 %Pegar caixa -> ponto de espera
    X=0;
    Y=coordenadas_pol(2500,2050.15,t-34,3);
    Z=907.64;
    alfa=0;
    beta=0;
    gama=deg2rad(90);
end
    
if t>=37 && t<43 % Ponto espera -> pos circuferencia dist 2
    raio=2050.15; 
    %pos_final_traj=-1888.22;
    %ang_final_traj=abs(acos(pos_final_traj/raio_traj));
    ang_final_traj=2.7415;
    ang_inicial_traj=0;
    angulo=coordenadas_pol(ang_inicial_traj,ang_final_traj,t-37,6);
    Y=cos(angulo)*raio;
    X=sin(angulo)*raio;
    Z=907.64;
    alfa=0;
    beta=0;
    gama=coordenadas_pol(deg2rad(90),deg2rad(-90),t-37,6);
end 

if t>=43 && t<46 % Pos circuferencia dist2 -> 10mm do pallete dist 2
    X=coordenadas_pol(798.5410,800.15,t-43,3);
    Y=coordenadas_pol(-2040.39,-2049.85,t-43,3);
    Z=coordenadas_pol(907.64,255.64,t-43,3);
    alfa=0;
    beta=0;
    gama=deg2rad(-90);
end 

if t>=46 && t<48 %10mm do pallete dist 2 -> encaixe no pallete dist 2
    X=800.15;
    Y=-2049.85;
    Z=coordenadas_pol(255.64,245.64,t-46,2);
    alfa=0;
    beta=0;
    gama=deg2rad(-90);
end 

if t>=48 && t<50 %encaixe pallete dist 2 -> retraido caixa dist 2
    X=800.15;
    Y=coordenadas_pol(-2049.85,-1899.85,t-48,2);
    Z=245.64;
    alfa=0;
    beta=0;
    gama=deg2rad(-90);
end 
    
if t>=50 && t<53 %retraido caixa dist 2 -> pos circuferencia dist 2
    X=coordenadas_pol(800.15,798.58,t-50,3);
    Y=coordenadas_pol(-1899.85,-1888.22,t-50,3);
    Z=coordenadas_pol(245.64,907.64,t-50,3);
    alfa=0;
    beta=0;
    gama=deg2rad(-90);
end 

if t>=53 && t<59 %pos circuferencia dist 2 -> ponto de espera
    raio=2050.15; 
    ang_inicial_traj=2.7415;
    ang_final_traj=0;
    angulo=coordenadas_pol(ang_inicial_traj,ang_final_traj,t-53,6);
    Y=cos(angulo)*raio;
    X=sin(angulo)*raio;
    Z=907.64;
    alfa=0;
    beta=0;
    gama=coordenadas_pol(deg2rad(-90),deg2rad(90),t-53,6);
end 

if t>=59 && t<62 %ponto de espera -> pegar caixa
    X=0;
    Y=coordenadas_pol( 2050.15,2500,t-59,3);
    Z=907.64;
    alfa=0;
    beta=0;
    gama=deg2rad(90);
end 

if t>=62 && t<65 % Pegar caixa -> Ponto de Espera
    X=coordenadas_pol(0,0,t-62,3);
    Y=coordenadas_pol(2500,2050.15,t-62,3);
    Z=coordenadas_pol(907.64,907.64,t-62,3);
    alfa=0;
    beta=0;
    gama=deg2rad(90);
end 

if t>=65 && t<71 %Ponto de espera ->Pós Circunferência
    raio=2050.15; 
    ang_final_traj=3.044;
    ang_inicial_traj=0;
    angulo=coordenadas_pol(ang_inicial_traj,ang_final_traj,t-65,6);
    Y=cos(angulo)*raio;
    X=sin(angulo)*raio;
    Z=907.64;
    alfa=0;
    beta=0;
    gama=coordenadas_pol(deg2rad(90),deg2rad(-90),t-65,6);
end 

if t>=71 && t<74 %Pos circuferencia -> (10mm do pallet)
    X=coordenadas_pol(199.7621,199.85,t-71,3);
    Y=coordenadas_pol(-2040.39,-2049.85,t-71,3);
    Z=coordenadas_pol(907.64,595.64,t-71,3);
    alfa=0;
    beta=0;
    gama=deg2rad(-90);
end 

if t>=74 && t<76 %10mm pallete -> (Encaixe no pallet)
    X=199.85;
    Y=-2049.85;
    Z=coordenadas_pol(595.64,585.64,t-74,2);
    alfa=0;
    beta=0;
    gama=deg2rad(-90);
end 

if t>=76 && t<78 %Encaixe pallet -> (Retraído em Y da Caixa)
    X=199.85;
    Y=coordenadas_pol(-2049.85,-1899.85,t-76,2);
    Z=585.64;
    alfa=0;
    beta=0;
    gama=deg2rad(-90);
end 
    
if t>=78 && t<81 %Retraido y caixa -> (Pós Circunferência)
    X=199.85;
    Y=coordenadas_pol(-1899.85,-2040.39,t-78,3);
    Z=coordenadas_pol(585.64,907.64,t-78,3);
    alfa=0;
    beta=0;
    gama=deg2rad(-90);
end 

if t>=81 && t<87 %Pós circuferência -> (Ponto de Espera)
    raio=2050.15; 
    ang_inicial_traj=3.044;
    ang_final_traj=0;
    angulo=coordenadas_pol(ang_inicial_traj,ang_final_traj,t-81,6);
    Y=cos(angulo)*raio;
    X=sin(angulo)*raio;
    Z=907.64;
    alfa=0;
    beta=0;
    gama=coordenadas_pol(deg2rad(-90),deg2rad(90),t-81,6); 
end 
if t>=87 && t<90 %ponto de espera -> (Pega a Caixa)
    X=0;
    Y=coordenadas_pol(2050.15,2500,t-87,3);
    Z=907.64;
    alfa=0;
    beta=0;
    gama=deg2rad(90);
end 
if t>=90 && t<93  %pega caixa -> (Ponto de Espera)
    X=0;
    Y=coordenadas_pol(2500,2050.15,t-90,3);
    Z=907.64;
    alfa=0;
    beta=0;
    gama=deg2rad(90);
end 
if t>=93 && t<99 %ponto espera ->(Pós Circunferência)
    raio=2050.15; 
    %pos_final_traj=-1888.22;
    %ang_final_traj=abs(acos(pos_final_traj/raio_traj));
    ang_final_traj=2.7415;
    ang_inicial_traj=0;
    angulo=coordenadas_pol(ang_inicial_traj,ang_final_traj,t-93,6);
    Y=cos(angulo)*raio;
    X=sin(angulo)*raio;
    Z=907.64;
    alfa=0;
    beta=0;
    gama=coordenadas_pol(deg2rad(90),deg2rad(-93),t-93,6);
end 
if t>=99 && t<102 %pos circuferencia -> (10mm do pallet)
    X=coordenadas_pol(798.541,800.15,t-99,3);
    Y=coordenadas_pol(-1888.22,-2049.85,t-99,3);
    Z=907.64;
    alfa=0;
    beta=0;
    gama=deg2rad(-90);
end
if t>=102 && t<104 %10mm palete -> (Encaixe no pallet)
    X=800.15;
    Y=-2049.85;
    Z=coordenadas_pol(595.64,585.64,t-102,2);
    alfa=0;
    beta=0;
    gama=deg2rad(-90);
end
if t>=104 && t<106 %encaixe pallete -> (Retraído em Y da Caixa)
    X=800.15;
    Y=coordenadas_pol(-2049.85,-1899.85,t-104,2);
    Z=coordenadas_pol(585.64,585.64,t-104,2);
    alfa=0;
    beta=0;
    gama=deg2rad(-90);
end
if t>=106 && t<109 %retraido caixa -> (Pós Circunferência)
    X=coordenadas_pol(800.15,798.541,t-106,3);
    Y=coordenadas_pol(-1899.85,-1888.22,t-106,3);
    Z=coordenadas_pol(585.64,907.64,t-106,3);
    alfa=0;
    beta=0;
    gama=deg2rad(-90);
end
if t>=109 %&& t=<115 %pos circ -> (Ponto de Espera)
    raio=2050.15; 
    ang_inicial_traj=2.7415;
    ang_final_traj=0;
    angulo=coordenadas_pol(ang_inicial_traj,ang_final_traj,t-109,6);
    Y=cos(angulo)*raio;
    X=sin(angulo)*raio;
    Z=907.64;
    alfa=0;
    beta=0;
    gama=coordenadas_pol(deg2rad(-90),deg2rad(90),t-109,6);
end

X=X/1000;
Y=Y/1000;
Z=Z/1000;
tarefa=[X,Y,Z,alfa,beta,gama];
end
